simulink model "Substation"  (R2023a)
settings: Solver=ode23tb  StartTime=0.0  StopTime=50  MaxStep=0.066666666666666671  RelTol=1e-4  EnableMultiTasking=on
undefined symbols (not defined in the file): D11, Delta
libraries: dspnetwork x14, spsMultimeterLib x4, dspstat3 x4, spsThreePhaseBreakerLib x4, spsThreePhaseFaultLib x4, spsThreePhaseSeriesRLCLoadLib x1, spsThreePhaseTransformerTwoWindingsLib x1, spsThreePhaseVIMeasurementLib x1, spsThreePhaseSourceLib x1, sps_lib x1
settings Model: PacingRate=10  Creator=ahelmasry  LastModifiedBy=hbku
settings SolverCC: ZeroCrossControl=EnableAll  ZeroCrossAlgorithm=Adaptive  AlgebraicLoopSolver=TrustRegion  SolverResetMethod=Robust
settings DataIOCC: LimitDataPoints=on  SaveFormat=Array  ReturnWorkspaceOutputs=off
settings OptimizationCC: ReuseModelBlockBuffer=off  ExpressionDepthLimit=2147483647  LifeSpan=inf
settings DebuggingCC: UnderspecifiedInitializationDetection=Classic  MergeDetectMultiDrivingBlocksExec=none  MaskedZcDiagnostic=none  IgnoredZcDiagnostic=none  SolverPrmCheckMsg=warning  FcnCallInpInsideContextMsg=warning  StateNameClashWarn=warning  SFUnexpectedBacktrackingDiag=warning  SFNoUnconditionalDefaultTransitionDiag=warning  SFExecutionAtInitializationDiag=none  ArithmeticOperatorsInVariantConditions=warning
settings HardwareCC: ProdBitPerPointer=32  ProdBitPerSizeT=32  ProdBitPerPtrDiffT=32  ProdLargestAtomicFloat=None  ProdIntDivRoundTo=Undefined  ProdEndianess=Unspecified  ProdWordSize=32  ProdHWDeviceType=32-bit Generic
settings ModelReferenceCC: EnableRefExpFcnMdlSchedulingChecks=on  PropagateSignalLabelsOutOfModel=off
settings SFSimCC: SimUseLocalCustomCode=off  CustomCodeUndefinedFunction=UseInterfaceOnly
settings RTWCC: RTWUseLocalCustomCode=off
settings CodeAppCC: StateflowObjectComments=on
settings GRTTargetCC: TargetLangStandard=C89/C90 (ANSI)  CombineOutputUpdateFcns=off  GRTInterface=on
settings ConfigComp: CovMetricSettings=dw  CovSaveCumulativeToWorkspaceVar=on  CovSaveSingleToWorkspaceVar=on  CovExternalEMLEnable=off

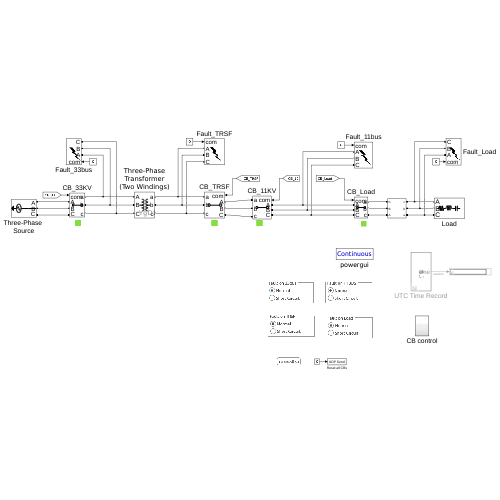
[thumbnail: Simulink's stored preview of the top-level diagram]
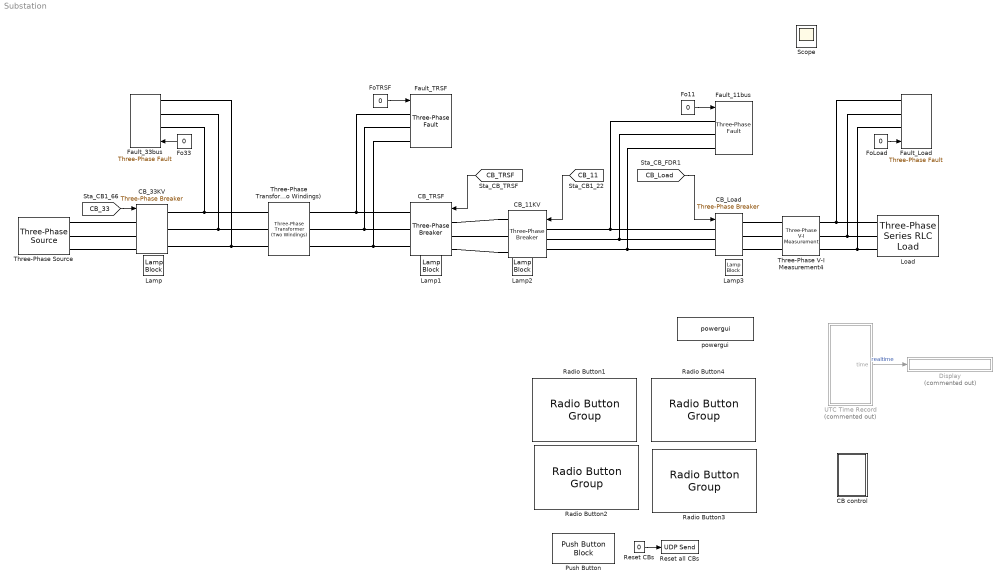
== system Substation ==
  CB control : Subsystem
  CB_11KV : spsThreePhaseBreakerLib/Three-Phase Breaker  InitialState=closed  SwitchA=on  SwitchB=on  SwitchC=on  SwitchTimes="[1/10  2/10]"  External=on  BreakerResistance=0.0001  SnubberResistance=inf  SnubberCapacitance=inf  Measurements=Breaker voltages and currents
  CB_33KV : spsThreePhaseBreakerLib/Three-Phase Breaker  InitialState=closed  SwitchA=on  SwitchB=on  SwitchC=on  SwitchTimes="[1/10  2/10]"  External=on  BreakerResistance=0.0001  SnubberResistance=inf  SnubberCapacitance=inf  Measurements=Breaker voltages and currents
  CB_Load : spsThreePhaseBreakerLib/Three-Phase Breaker  InitialState=closed  SwitchA=on  SwitchB=on  SwitchC=on  SwitchTimes="[1/10  2/10]"  External=on  BreakerResistance=0.0001  SnubberResistance=inf  SnubberCapacitance=inf  Measurements=Breaker voltages and currents
  CB_TRSF : spsThreePhaseBreakerLib/Three-Phase Breaker  InitialState=closed  SwitchA=on  SwitchB=on  SwitchC=on  SwitchTimes="[1/10  2/10]"  External=on  BreakerResistance=0.0001  SnubberResistance=inf  SnubberCapacitance=inf  Measurements=Breaker voltages and currents
  Display : Display  Commented=on
  Fault_11bus : spsThreePhaseFaultLib/Three-Phase Fault  InitialStates=0  FaultA=on  FaultB=on  FaultC=on  GroundFault=off  SwitchTimes="[1/60  5/60]"  External=on  SwitchStatus=NaN  FaultResistance=0.0001  GroundResistance=0.01  SnubberResistance=inf  SnubberCapacitance=inf  Measurements=Fault voltages and currents
  Fault_33bus : spsThreePhaseFaultLib/Three-Phase Fault  InitialStates=0  FaultA=on  FaultB=on  FaultC=on  GroundFault=off  SwitchTimes="[1/60  5/60]"  External=on  SwitchStatus=NaN  FaultResistance=0.0001  GroundResistance=0.01  SnubberResistance=inf  SnubberCapacitance=inf  Measurements=Fault voltages and currents
  Fault_Load : spsThreePhaseFaultLib/Three-Phase Fault  InitialStates=0  FaultA=on  FaultB=on  FaultC=on  GroundFault=off  SwitchTimes="[1/60  5/60]"  External=on  SwitchStatus=NaN  FaultResistance=0.0001  GroundResistance=0.00001  SnubberResistance=inf  SnubberCapacitance=inf  Measurements=Fault voltages and currents
  Fault_TRSF : spsThreePhaseFaultLib/Three-Phase Fault  InitialStates=0  FaultA=on  FaultB=on  FaultC=on  GroundFault=off  SwitchTimes="[1/60  5/60]"  External=on  SwitchStatus=NaN  FaultResistance=0.0001  GroundResistance=0.01  SnubberResistance=inf  SnubberCapacitance=inf  Measurements=Fault voltages and currents
  Fo11 : Constant  Value=0  SampleTime=0
  Fo33 : Constant  Value=0  SampleTime=0
  FoLoad : Constant  Value=0  SampleTime=0
  FoTRSF : Constant  Value=0  SampleTime=0
  Lamp{,1..3} (4 alike) : LampBlock  LabelPosition=Hide  Icon=Square
  Load : spsThreePhaseSeriesRLCLoadLib/Three-Phase Series RLC Load  LConnTagsString=A|B|C  Configuration=Delta  NominalVoltage=11000  Vabc=[1e3 1e3 1e3]  Vabcp=[1e3 1e3 1e3]  NominalFrequency=50  UnbalancedPower=off  ActivePower=1e6  InductivePower=100  CapacitivePower=100  Pabc=[10e3 9e3 11e3]  QLabc=[100 90 110]  QCabc=[100 90 110]  Pabcp=[10e3 9e3 11e3]  QLabcp=[100 90 110]  QCabcp=[100 90 110]  Measurements=Branch voltages and currents  LoadType=constant Z
  Push Button : PushButtonBlock  ButtonText=Reset All CBs  OffValue=0.000000
  Radio Button1 : RadioButtonGroup  LabelPosition=Hide  SelectedLabel=Normal  ButtonGroupName=Fault on 33bus
      settings: Values={{'Normal', 'Short Circuit'}, [0 1]}
  Radio Button2 : RadioButtonGroup  LabelPosition=Hide  SelectedLabel=Normal  ButtonGroupName=Fault on TRSF
      settings: Values={{'Normal', 'Short Circuit'}, [0 1]}
  Radio Button3 : RadioButtonGroup  LabelPosition=Hide  SelectedLabel=Normal  ButtonGroupName=Fault on Load
      settings: Values={{'Normal', 'Short Circuit'}, [0 1]}
  Radio Button4 : RadioButtonGroup  LabelPosition=Hide  SelectedLabel=Normal  ButtonGroupName=Fault on 11BUS
      settings: Values={{'Normal', 'Short Circuit'}, [0 1]}
  Reset CBs : Constant  Value=0  SampleTime=0
  Reset all CBs : dspnetwork/UDP Send  remoteURL='23.23.23.255'  remotePort=10000  localURL='0.0.0.0'  localPortSource=Automatically determine  localPort=-1  sendBufferSize=8192  sampletime=-1  blockPlatform=[]  separateLengthPort=0
  Three-Phase Transformer (Two Windings) : spsThreePhaseTransformerTwoWindingsLib/Three-Phase Transformer (Two Windings)  Winding1Connection=Yg  Winding2Connection=Delta (D11)  CoreType=Three single-phase transformers  SetSaturation=off  Hysteresis=off  DataFile='hysteresis'  SetInitialFlux=off  Measurements=All measurements (V I Fluxes)  UNITS=pu  NominalPower=[ 25e6 , 50 ]  Winding1=[ 33e3 , 0.002 , 0.08 ]  Winding2=[ 11e3 , 0.002 , 0.08 ]  Rm=500  Lm=500  L0=0.5  Saturation=[ 0,0 ; 0.0024,1.2 ; 1.0,1.52 ]  InitialFluxes=[0.79999 -0.79999 0.69999]  BreakLoop=off  DiscreteSolver=Trapezoidal iterative  DataType=off  TransfoNumber=1
  Three-Phase V-I Measurement4 : spsThreePhaseVIMeasurementLib/Three-Phase V-I Measurement  VoltageMeasurement=phase-to-phase  SetLabelV=on  LabelV=Vfdr1  Vpu=off  VpuLL=off  CurrentMeasurement=yes  SetLabelI=on  LabelI=Ifdr1  Ipu=off  Pbase=100e6  Vbase=500e3  OutputType=Complex  PhasorSimulation=off  PSBequivalent=0
  Three-Phase Source : spsThreePhaseSourceLib/Three-Phase Source  InternalConnection=Yg  VoltagePhases=off  Voltage=33000  PhaseAngle=120  Voltage_phases=[66000 66000 66000]  PhaseAngles_phases=[0 -120 +120]  Frequency=50  NonIdealSource=off  SpecifyImpedance=off  Resistance=0.8929  Inductance=16.58e-3  ShortCircuitLevel=100e6  BaseVoltage=25e3  XRratio=7  BusType=swing  Pref=10e3  Qref=0  Prefabc=[10e3, 10e3, 10e3]  Qrefabc=[0, 0, 0]  Qmin=-inf  Qmax=inf
  UTC Time Record : MATLAB Function  Commented=on  TreatAsAtomicUnit=on
  powergui : sps_lib/powergui  Priority=1  SimulationMode=Continuous  SampleTime=50e-6  frequency=50  Iterations=50  frequencyindice=50  Pbase=100e6  ErrMax=1e-4  UnitsV=kV  UnitsW=MW  buscounter=0  FunctionMessages=off  echomessages=off  EnableUseOfTLC=off  CurrentSourceSwitches=off  DisableSnubberDevices=off  DisableRonSwitches=off  DisableVfSwitches=off  DisplayEquations=off  AutomaticDiscreteSolvers=off  SolverType=Tustin/Backward Euler (TBE)  Interpol=off  ExternalGateDelay=off  methode=off  Ts=100  x0status=blocks  SPID=off  SwTol=0  HookPort=off  NonlinearTolerance=1e-4  nMaxIteration=100  ContinueOnMaxIteration=off  RestoreLinks=warning  ResistiveCurrentMeasurement=off  Frange=[0:2:500]  Ylog=off  Xlog=on  ShowGrid=off  save=off  variable=ZData  structure=0  ZoomFFT=off  StartTime=0.0  cycles=1  DisplayStyle=1  fundamental=60  FreqAxis=off  MaxFrequency=1000  frequencyindicesteady=1  RmsSteady=1  display=off
  Scope : Scope
  wires:
  FoTRSF/1 -> Fault_TRSF/1
  [CB_33] -> CB_33KV/1
  [CB_TRSF] -> CB_TRSF/1
  [CB_Load] -> CB_Load/1
  Fo11/1 -> Fault_11bus/1
  FoLoad/1 -> Fault_Load/1
  Fo33/1 -> Fault_33bus/1
  [CB_11] -> CB_11KV/1
  UTC Time Record/1(time) -> Display/1  "realtime"
  Reset CBs/1 -> Reset all CBs/1
  connections:
  CB_11KV/RConn3 -- CB_TRSF/LConn3
  CB_11KV/RConn2 -- CB_TRSF/LConn2
  CB_11KV/RConn1 -- CB_TRSF/LConn1
  CB_33KV/RConn3 -- Fault_33bus/LConn3 -- Three-Phase Transformer (Two Windings)/LConn3
  Fault_33bus/LConn2 -- CB_33KV/RConn2 -- Three-Phase Transformer (Two Windings)/LConn2
  Fault_33bus/LConn1 -- CB_33KV/RConn1 -- Three-Phase Transformer (Two Windings)/LConn1
  CB_TRSF/RConn3 -- Fault_TRSF/LConn3 -- Three-Phase Transformer (Two Windings)/RConn3
  CB_TRSF/RConn2 -- Fault_TRSF/LConn2 -- Three-Phase Transformer (Two Windings)/RConn2
  CB_TRSF/RConn1 -- Fault_TRSF/LConn1 -- Three-Phase Transformer (Two Windings)/RConn1
  CB_33KV/LConn3 -- Three-Phase Source/RConn3
  CB_33KV/LConn2 -- Three-Phase Source/RConn2
  CB_33KV/LConn1 -- Three-Phase Source/RConn1
  Three-Phase V-I Measurement4/LConn2 -- CB_Load/RConn2
  Load/LConn2 -- Fault_Load/LConn2 -- Three-Phase V-I Measurement4/RConn2
  Three-Phase V-I Measurement4/LConn1 -- CB_Load/RConn3
  Three-Phase V-I Measurement4/LConn3 -- CB_Load/RConn1
  Load/LConn1 -- Fault_Load/LConn3 -- Three-Phase V-I Measurement4/RConn3
  Load/LConn3 -- Three-Phase V-I Measurement4/RConn1 -- Fault_Load/LConn1
  CB_11KV/LConn1 -- CB_Load/LConn1 -- Fault_11bus/LConn1
  CB_11KV/LConn2 -- CB_Load/LConn2 -- Fault_11bus/LConn2
  CB_11KV/LConn3 -- CB_Load/LConn3 -- Fault_11bus/LConn3

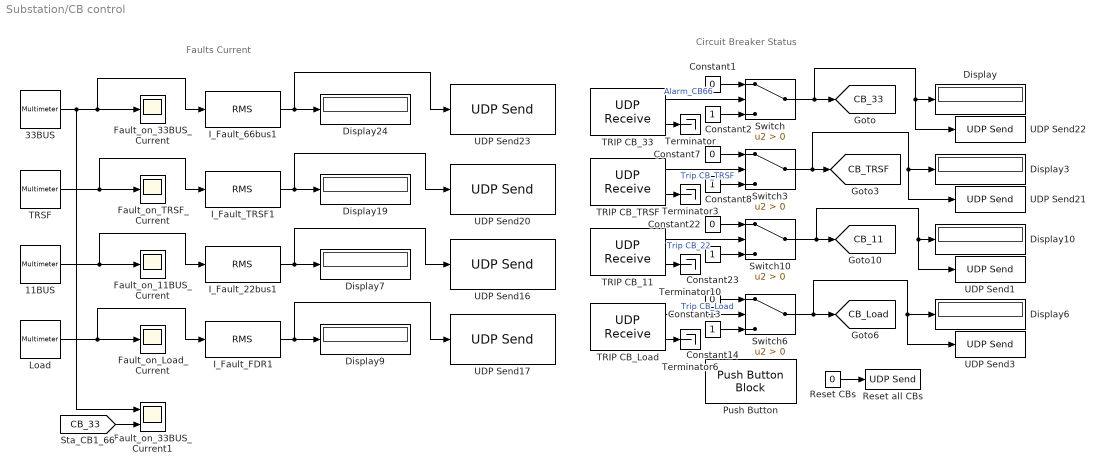
== system Substation/CB control ==
  note: Circuit Breaker Status
  note: Faults Current
  11BUS : spsMultimeterLib/Multimeter  L=75  sel=[49 50 51]  yselected={}  Gain=[1 1 1]  OutputType=Complex  PlotAtSimulationStop=off  PhasorSimulation=off
  33BUS : spsMultimeterLib/Multimeter  L=75  sel=[52 53 54]  yselected={}  Gain=[1 1 1]  OutputType=Complex  PlotAtSimulationStop=off  PhasorSimulation=off
  Constant{1,7,13,22} (4 alike) : Constant  Value=0
  Constant{2,8,14,23} (4 alike) : Constant
  Display{,3,6..7,9..10,19,24} (8 alike) : Display
  Fault_on_11BUS_Current : Scope
  Fault_on_33BUS_Current : Scope
  Fault_on_33BUS_Current1 : Scope  NumInputPorts=2
  Fault_on_Load_Current : Scope
  Fault_on_TRSF_Current : Scope
  I_Fault_22bus1 : dspstat3/RMS  run=off  directionMode=Specified dimension  dimension=1  reset_popup=None
  I_Fault_66bus1 : dspstat3/RMS  run=off  directionMode=Specified dimension  dimension=1  reset_popup=None
  I_Fault_FDR1 : dspstat3/RMS  run=off  directionMode=Specified dimension  dimension=1  reset_popup=None
  I_Fault_TRSF1 : dspstat3/RMS  run=off  directionMode=Specified dimension  dimension=1  reset_popup=None
  Load : spsMultimeterLib/Multimeter  L=75  sel=[55 56 57]  yselected={}  Gain=[1 1 1]  OutputType=Complex  PlotAtSimulationStop=off  PhasorSimulation=off
  Push Button : PushButtonBlock  ButtonText=Reset All CBs  OffValue=0.000000
  Reset CBs : Constant  Value=0  SampleTime=0
  Reset all CBs : dspnetwork/UDP Send  remoteURL='23.23.23.255'  remotePort=10000  localURL='0.0.0.0'  localPortSource=Automatically determine  localPort=-1  sendBufferSize=8192  sampletime=-1  blockPlatform=[]  separateLengthPort=0
  Switch{,3,6,10} (4 alike) : Switch  Criteria=u2 > Threshold  SaturateOnIntegerOverflow=off  InputSameDT=off
  TRIP CB_11 : dspnetwork/UDP Receive  localURL='0.0.0.0'  localPort=20111  remoteURL='23.23.23.0'  remotePort=-1  recvBufferSize=2  dims=1  signalDatatype=uint16  isComplex=off  isVarSize=off  showBlockingTime=off  blockingTime=0  sampletime=0  blockPlatform=[]
  TRIP CB_33 : dspnetwork/UDP Receive  localURL='0.0.0.0'  localPort=20133  remoteURL='23.23.23.0'  remotePort=-1  recvBufferSize=2  dims=1  signalDatatype=uint16  isComplex=off  isVarSize=off  showBlockingTime=off  blockingTime=0  sampletime=0  blockPlatform=[]
  TRIP CB_Load : dspnetwork/UDP Receive  localURL='0.0.0.0'  localPort=20100  remoteURL='23.23.23.0'  remotePort=-1  recvBufferSize=2  dims=1  signalDatatype=uint16  isComplex=off  isVarSize=off  showBlockingTime=off  blockingTime=0  sampletime=0  blockPlatform=[]
  TRIP CB_TRSF : dspnetwork/UDP Receive  localURL='0.0.0.0'  localPort=20122  remoteURL='23.23.23.0'  remotePort=-1  recvBufferSize=2  dims=1  signalDatatype=uint16  isComplex=off  isVarSize=off  showBlockingTime=off  blockingTime=0  sampletime=0  blockPlatform=[]
  TRSF : spsMultimeterLib/Multimeter  L=75  sel=[58 59 60]  yselected={}  Gain=[1 1 1]  OutputType=Complex  PlotAtSimulationStop=off  PhasorSimulation=off
  Terminator{,3,6,10} (4 alike) : Terminator
  UDP Send1 : dspnetwork/UDP Send  remoteURL='23.23.23.255'  remotePort=10111  localURL='0.0.0.0'  localPortSource=Automatically determine  localPort=-1  sendBufferSize=8192  sampletime=-1  blockPlatform=[]  separateLengthPort=0
  UDP Send16 : dspnetwork/UDP Send  remoteURL='23.23.23.255'  remotePort=30111  localURL='0.0.0.0'  localPortSource=Automatically determine  localPort=-1  sendBufferSize=8192  sampletime=-1  blockPlatform=[]  separateLengthPort=0
  UDP Send17 : dspnetwork/UDP Send  remoteURL='23.23.23.255'  remotePort=30100  localURL='0.0.0.0'  localPortSource=Automatically determine  localPort=-1  sendBufferSize=8192  sampletime=-1  blockPlatform=[]  separateLengthPort=0
  UDP Send20 : dspnetwork/UDP Send  remoteURL='23.23.23.255'  remotePort=30122  localURL='0.0.0.0'  localPortSource=Automatically determine  localPort=-1  sendBufferSize=8192  sampletime=-1  blockPlatform=[]  separateLengthPort=0
  UDP Send21 : dspnetwork/UDP Send  remoteURL='23.23.23.255'  remotePort=10122  localURL='0.0.0.0'  localPortSource=Automatically determine  localPort=-1  sendBufferSize=8192  sampletime=-1  blockPlatform=[]  separateLengthPort=0
  UDP Send22 : dspnetwork/UDP Send  remoteURL='23.23.23.255'  remotePort=10133  localURL='0.0.0.0'  localPortSource=Automatically determine  localPort=-1  sendBufferSize=8192  sampletime=-1  blockPlatform=[]  separateLengthPort=0
  UDP Send23 : dspnetwork/UDP Send  remoteURL='23.23.23.255'  remotePort=30133  localURL='0.0.0.0'  localPortSource=Automatically determine  localPort=-1  sendBufferSize=8192  sampletime=-1  blockPlatform=[]  separateLengthPort=0
  UDP Send3 : dspnetwork/UDP Send  remoteURL='23.23.23.255'  remotePort=10100  localURL='0.0.0.0'  localPortSource=Automatically determine  localPort=-1  sendBufferSize=8192  sampletime=-1  blockPlatform=[]  separateLengthPort=0
  tag scope: CB_11=global, CB_33=global, CB_Load=global, CB_TRSF=global
  wires:
  TRIP CB_TRSF/1 -> Switch3/2  "Trip CB_TRSF"
  Constant8/1 -> Switch3/3
  TRIP CB_Load/2 -> Terminator6/1
  TRIP CB_TRSF/2 -> Terminator3/1
  Constant2/1 -> Switch/3
  TRIP CB_33/1 -> Switch/2  "Alarm_CB66"
  Constant13/1 -> Switch6/1
  TRIP CB_33/2 -> Terminator/1
  Constant7/1 -> Switch3/1
  Constant14/1 -> Switch6/3
  Constant1/1 -> Switch/1
  Reset CBs/1 -> Reset all CBs/1
  Constant22/1 -> Switch10/1
  Constant23/1 -> Switch10/3
  Switch6/1 -> UDP Send3/1, Display6/1, [CB_Load]
  Switch10/1 -> UDP Send1/1, Display10/1, [CB_11]
  TRIP CB_11/1 -> Switch10/2  "Trip CB_22"
  TRIP CB_Load/1 -> Switch6/2  "Trip CB_Load"
  TRIP CB_11/2 -> Terminator10/1
  I_Fault_66bus1/1 -> UDP Send23/1, Display24/1
  Load/1 -> I_Fault_FDR1/1, Fault_on_Load_Current/1
  33BUS/1 -> Fault_on_33BUS_Current1/1, I_Fault_66bus1/1, Fault_on_33BUS_Current/1
  TRSF/1 -> I_Fault_TRSF1/1, Fault_on_TRSF_Current/1
  I_Fault_FDR1/1 -> UDP Send17/1, Display9/1
  I_Fault_22bus1/1 -> UDP Send16/1, Display7/1
  I_Fault_TRSF1/1 -> UDP Send20/1, Display19/1
  11BUS/1 -> I_Fault_22bus1/1, Fault_on_11BUS_Current/1
  Switch/1 -> UDP Send22/1, Display/1, [CB_33]
  Switch3/1 -> Display3/1, UDP Send21/1, [CB_TRSF]
  [CB_33] -> Fault_on_33BUS_Current1/2

== matlab function Substation/UTC Time Record ==
  data: time output
function time  = fcn

   eml.extrinsic('datetime');
   eml.extrinsic('posixtime');


   time = 0;

   [time] = posixtime(datetime('now', 'TimeZone','local'));
end
